simulink model "solar"  (R2021a)
settings: Solver=ode4  StartTime=0.0  StopTime=2  RelTol=1e-3
libraries: spsSeriesRLCBranchLib x3, spsVoltageMeasurementLib x2, spspowerguiLib x1, spsCurrentMeasurementLib x1, spsDiodeLib x1, spsIdealSwitchLib x1, simulink_extras x1, spsPVArrayLib x1, simulink x1, spsVariableResistorLib x1
settings Model: Creator=aks  LastModifiedBy=aks
settings SolverCC: ZeroCrossControl=DisableAll
settings DataIOCC: Refine=100

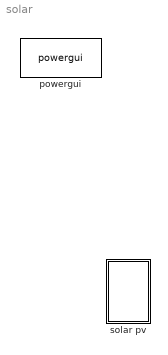
== system solar ==
  powergui : spspowerguiLib/powergui  Priority=1  SimulationMode=Discrete  SampleTime=1e-6  frequency=60  Iterations=50  frequencyindice=0  Pbase=100e6  ErrMax=1e-4  UnitsV=kV  UnitsW=MW  buscounter=0  FunctionMessages=off  echomessages=off  EnableUseOfTLC=off  CurrentSourceSwitches=off  DisableSnubberDevices=off  DisableRonSwitches=off  DisableVfSwitches=off  DisplayEquations=off  AutomaticDiscreteSolvers=off  SolverType=Tustin/Backward Euler (TBE)  Interpol=off  ExternalGateDelay=off  methode=off  Ts=100  x0status=blocks  SPID=on  SwTol=0  HookPort=off  NonlinearTolerance=1e-4  nMaxIteration=100  ContinueOnMaxIteration=off  RestoreLinks=warning  ResistiveCurrentMeasurement=off  Frange=[0:2:500]  Ylog=off  Xlog=on  ShowGrid=off  save=off  variable=ZData  structure=0  ZoomFFT=off  StartTime=0.0  cycles=1  DisplayStyle=1  fundamental=60  FreqAxis=off  MaxFrequency=1000  frequencyindicesteady=1  RmsSteady=1  display=off
  solar pv : Subsystem

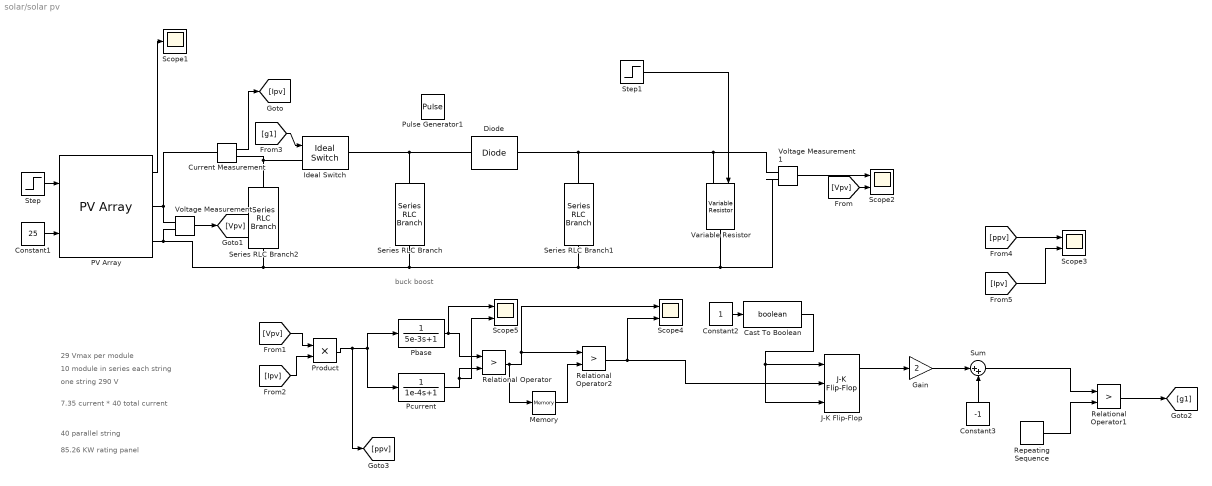
== system solar/solar pv ==
  note: buck boost
  note: 85.26 KW rating panel
  note: 40 parallel string
  note: 7.35 current * 40 total current
  note: one string 290 V
  note: 10 module in series each string
  note: 29 Vmax per module
  Cast To Boolean : DataTypeConversion  OutDataTypeStr=boolean
  Constant1 : Constant  Value=25
  Constant2 : Constant
  Constant3 : Constant  Value=-1
  Current Measurement : spsCurrentMeasurementLib/Current Measurement  PhasorSimulation=off  OutputType=Complex  PSBequivalent=0
  Diode : spsDiodeLib/Diode  Ron=1e-5  Lon=0  Vf=0.8  IC=0  UseSnubber=0  Rs=500  Cs=250e-9  Measurements=off
  Gain : Gain  Gain=2
  Ideal Switch : spsIdealSwitchLib/Ideal Switch  Ron=0.001  Lon=0  IC=0  Rs=1e5  Cs=inf  Measurements=off
  J-K Flip-Flop : simulink_extras/Flip Flops/J-K Flip-Flop  initial_condition=1
  Memory : Memory  InheritSampleTime=on
  PV Array : spsPVArrayLib/PV Array  Npar=40  Nser=10  PlotType=array @ 1000 W/m2 & specified temperatures  S_vec="[ 1000  500  100 ]"  Temp_C_vec=[ 45 25]  ModuleName=User-defined  PlotWhenSelected=off  Pm=213.15  Ncell=60  Voc=36.3  Isc=7.84  Vm=29  Im=7.35  beta_Voc_pc=-0.36099  alpha_Isc_pc=0.102  beta_Voc=-0.13104  alpha_Isc=0.0079968  IL=7.8654  I0=2.9273e-10  nI=0.98119  Rsh=313.0553  Rs=0.39381  RobustModel=off  RobustCellTemperature=313.3991  BAL=on  Tc=1e-6  Tfilter=5e-5
  Pbase : TransferFcn  Denominator=[5e-3 1]
  Pcurrent : TransferFcn  Denominator=[1e-4 1]
  Product : Product
  Pulse Generator1 : DiscretePulseGenerator  PulseType=Time based  Period=1/10e3  PulseWidth=90
  Relational Operator : RelationalOperator  Operator=>  OutDataTypeStr=boolean  RndMeth=Simplest
  Relational Operator1 : RelationalOperator  Operator=>  OutDataTypeStr=boolean  RndMeth=Simplest
  Relational Operator2 : RelationalOperator  Operator=>  OutDataTypeStr=boolean  RndMeth=Simplest
  Repeating Sequence : simulink/Sources/Repeating Sequence  rep_seq_t=[0 1/40e3 1/20e3 3/40e3 1/10e3]  rep_seq_y=[0 1 0 -1 0]
  Scope1 : Scope
  Scope{2..5} (4 alike) : Scope  NumInputPorts=2
  Series RLC Branch : spsSeriesRLCBranchLib/Series RLC Branch  LConnTagsString=__new0  RConnTagsString=__new0  BranchType=L  Resistance=1  Inductance=10e-3  SetiL0=off  InitialCurrent=0  Capacitance=1e-6  Setx0=off  InitialVoltage=0  Measurements=None
  Series RLC Branch1 : spsSeriesRLCBranchLib/Series RLC Branch  LConnTagsString=__new0  RConnTagsString=__new0  BranchType=C  Resistance=1  Inductance=1e-3  SetiL0=off  InitialCurrent=0  Capacitance=100e-6  Setx0=off  InitialVoltage=0  Measurements=None
  Series RLC Branch2 : spsSeriesRLCBranchLib/Series RLC Branch  LConnTagsString=__new0  RConnTagsString=__new0  BranchType=C  Resistance=1  Inductance=1e-3  SetiL0=off  InitialCurrent=0  Capacitance=100e-6  Setx0=off  InitialVoltage=0  Measurements=None
  Step : Step  Before=1000  After=1000  SampleTime=0
  Step1 : Step  Before=50  After=100  SampleTime=0
  Sum : Sum  Inputs=|++
  Variable Resistor : spsVariableResistorLib/Variable Resistor  Rabsmin=1e-3
      settings: SourceProductBaseCode=PS
  Voltage Measurement : spsVoltageMeasurementLib/Voltage Measurement  PhasorSimulation=off  OutputType=Complex  PSBequivalent=0
  Voltage Measurement1 : spsVoltageMeasurementLib/Voltage Measurement  PhasorSimulation=off  OutputType=Complex  PSBequivalent=0
  wires:
  Constant1/1 -> PV Array/2
  Step/1 -> PV Array/1
  PV Array/1 -> Scope1/1
  Current Measurement/1 -> [Ipv]
  Voltage Measurement/1 -> [Vpv]
  Voltage Measurement1/1 -> Scope2/1
  [Vpv] -> Scope2/2
  [Vpv] -> Product/1
  [Ipv] -> Product/2
  Pbase/1 -> Scope5/1, Relational Operator/1
  Pcurrent/1 -> Scope5/2, Relational Operator/2
  Constant2/1 -> Cast To Boolean/1
  Cast To Boolean/1 -> J-K Flip-Flop/3, J-K Flip-Flop/1
  J-K Flip-Flop/1 -> Gain/1
  Gain/1 -> Sum/1
  Constant3/1 -> Sum/2
  Repeating Sequence/1 -> Relational Operator1/2
  Relational Operator1/1 -> [g1]
  Product/1 -> [ppv], Pcurrent/1, Pbase/1
  [ppv] -> Scope3/1
  Relational Operator/1 -> Scope4/1, Relational Operator2/1, Memory/1
  Memory/1 -> Relational Operator2/2
  Relational Operator2/1 -> Scope4/2, J-K Flip-Flop/2
  [Ipv] -> Scope3/2
  [g1] -> Ideal Switch/1
  Sum/1 -> Relational Operator1/1
  Step1/1 -> Variable Resistor/1
  connections:
  PV Array/RConn1 -- Voltage Measurement/LConn1 -- Current Measurement/LConn1
  Series RLC Branch2/RConn1 -- Variable Resistor/RConn1 -- Voltage Measurement1/LConn2 -- Series RLC Branch1/RConn1 -- Series RLC Branch/RConn1 -- Voltage Measurement/LConn2 -- PV Array/RConn2
  Series RLC Branch/LConn1 -- Diode/RConn1 -- Ideal Switch/RConn1
  Series RLC Branch1/LConn1 -- Variable Resistor/LConn1 -- Voltage Measurement1/LConn1 -- Diode/LConn1
  Ideal Switch/LConn1 -- Series RLC Branch2/LConn1 -- Current Measurement/RConn1
